simulink library "cdsSwitch1"  (Simulink 6.2)
settings Model: LastModifiedBy=rolf

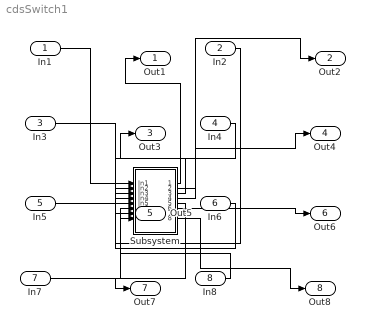
== system cdsSwitch1 ==
  In1 : Inport  Port=1  LatchInput=off
  In2 : Inport  Port=2  LatchInput=off
  In3 : Inport  Port=3  LatchInput=off
  In4 : Inport  Port=4  LatchInput=off
  In5 : Inport  Port=5  LatchInput=off
  In6 : Inport  Port=6  LatchInput=off
  In7 : Inport  Port=7  LatchInput=off
  In8 : Inport  Port=8  LatchInput=off
  Subsystem : Subsystem
  Out1 : Outport
  Out2 : Outport  Port=2
  Out3 : Outport  Port=3
  Out4 : Outport  Port=4
  Out5 : Outport  Port=5
  Out6 : Outport  Port=6
  Out7 : Outport  Port=7
  Out8 : Outport  Port=8
  wires:
  In1/1 -> Subsystem/1(In1)
  In2/1 -> Subsystem/2(In2)
  Subsystem/1(Out1) -> Out1/1
  Subsystem/2(Out2) -> Out2/1
  In3/1 -> Subsystem/3(In3)
  In4/1 -> Subsystem/4(In4)
  Subsystem/3(Out3) -> Out3/1
  Subsystem/4(Out4) -> Out4/1
  In5/1 -> Subsystem/5(In5)
  In6/1 -> Subsystem/6(In6)
  Subsystem/5(Out5) -> Out5/1
  Subsystem/6(Out6) -> Out6/1
  In7/1 -> Subsystem/7(In7)
  In8/1 -> Subsystem/8(In8)
  Subsystem/7(Out7) -> Out7/1
  Subsystem/8(Out8) -> Out8/1

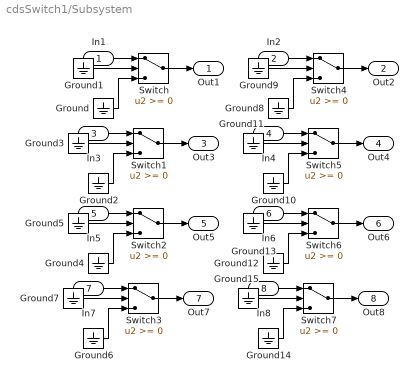
== system cdsSwitch1/Subsystem ==
  In1 : Inport  Port=1  LatchInput=off
  In2 : Inport  Port=2  LatchInput=off
  In3 : Inport  Port=3  LatchInput=off
  In4 : Inport  Port=4  LatchInput=off
  In5 : Inport  Port=5  LatchInput=off
  In6 : Inport  Port=6  LatchInput=off
  In7 : Inport  Port=7  LatchInput=off
  In8 : Inport  Port=8  LatchInput=off
  Ground{,1..15} (16 alike) : Ground
  Switch{,1..7} (8 alike) : Switch
  Out1 : Outport
  Out2 : Outport  Port=2
  Out3 : Outport  Port=3
  Out4 : Outport  Port=4
  Out5 : Outport  Port=5
  Out6 : Outport  Port=6
  Out7 : Outport  Port=7
  Out8 : Outport  Port=8
  wires:
  Switch7/1 -> Out8/1
  Switch3/1 -> Out7/1
  In8/1 -> Switch7/1
  In7/1 -> Switch3/1
  Switch6/1 -> Out6/1
  Switch2/1 -> Out5/1
  In6/1 -> Switch6/1
  In5/1 -> Switch2/1
  Switch5/1 -> Out4/1
  Switch1/1 -> Out3/1
  In4/1 -> Switch5/1
  In3/1 -> Switch1/1
  Switch4/1 -> Out2/1
  Switch/1 -> Out1/1
  In2/1 -> Switch4/1
  In1/1 -> Switch/1
  Ground15/1 -> Switch7/2
  Ground14/1 -> Switch7/3
  Ground13/1 -> Switch6/2
  Ground12/1 -> Switch6/3
  Ground11/1 -> Switch5/2
  Ground10/1 -> Switch5/3
  Ground9/1 -> Switch4/2
  Ground8/1 -> Switch4/3
  Ground7/1 -> Switch3/2
  Ground6/1 -> Switch3/3
  Ground5/1 -> Switch2/2
  Ground4/1 -> Switch2/3
  Ground3/1 -> Switch1/2
  Ground2/1 -> Switch1/3
  Ground1/1 -> Switch/2
  Ground/1 -> Switch/3
